simulink model "report01"  (R2019a)
settings: Solver=VariableStepAuto  StartTime=0.0  StopTime=10  RelTol=1e-3
settings Model: Creator=zgz  LastModifiedBy=zgz
settings DataIOCC: ReturnWorkspaceOutputs=off

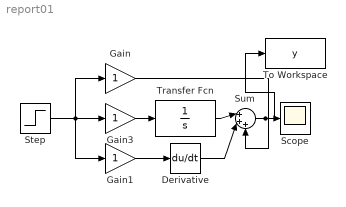
== system report01 ==
  Derivative : Derivative  CoefficientInTFapproximation=1
  Gain : Gain
  Gain1 : Gain
  Gain3 : Gain
  Scope : Scope
  Step : Step  SampleTime=0
  Sum : Sum  Inputs=|+++
  To Workspace : ToWorkspace  VariableName=y  SampleTime=-1
  Transfer Fcn : TransferFcn  Denominator=[1 0]
  wires:
  Step/1 -> Gain1/1, Gain3/1, Gain/1
  Gain3/1 -> Transfer Fcn/1
  Transfer Fcn/1 -> Sum/1
  Gain1/1 -> Derivative/1
  Derivative/1 -> Sum/2
  Sum/1 -> To Workspace/1, Scope/1
  Gain/1 -> Sum/3
